simulink model "MultiUAV_DroneShow"  (R2026a)
settings: Solver=ode1  StopTime=74.3333  FixedStep=Ts_sim  MaxStep=0.01  AbsTol=1e-6
PreLoadFcn:
  | setupParams
values from neighbouring files (symbols this model uses):
  arm_duration = 2    [setupParams.m]
  gnss_deny_mask = false(N_uav, 1)    [setupParams.m]
  gnss_err_gain = sqrt(1 - gnss_err_pole^2)    [setupParams.m]
  gnss_err_pole = exp(-Ts_sim / gnss_err_tau)    [setupParams.m]
  gnss_err_seed = reshape(40000 + (1:(N_uav * 3)), N_uav, 3)    [setupParams.m]
  gps_accuracy_rtk_fix = 0.02    [setupParams.m]
  gps_lock_duration = 2    [setupParams.m]
  gravity = 9.81    [setupParams.m]
  hb_period_ticks = mavlink_hb_interval / Ts_sim    (= 100)    [setupParams.m]
  init_positions = init_positions(pad_of, :)    [planShow.m]    (also in setupParams.m = plan.init_positions)
  Kd_pos = repmat([Kd_xy Kd_xy Kd_z], N_uav, 1)    [setupParams.m]
  Kff_pos = Kd_pos    [setupParams.m]
  Kp_pos = repmat([Kp_xy Kp_xy Kp_z], N_uav, 1)    [setupParams.m]
  land_end_time = plan.land_end_time    [packShowUpload.m]    (also in planShow.m = show_flight_duration + land_duration; setupParams.m)
  land_speed = cfg.land_speed    [planShow.m]
  land_start_time = show_flight_duration    [planShow.m]    (also in setupParams.m = plan.land_start_time)
  land_total_duration = land_duration + land_settle    [planShow.m]    (also in setupParams.m = plan.land_total_duration)
  mav_sys_span = 250    [setupParams.m]
  N_uav = 20    [DroneShowExample.m]    (also in packShowUpload.m = cfg.N_uav; planShow.m = cfg.N_uav; setupParams.m = 10)
  num_waypoints = length(upload_times)    [packShowUpload.m]    (also in setupParams.m = pack.num_waypoints)
  rtcm_data_bytes = 180    [setupParams.m]
  rtcm_interval = 1.0    (= 1)    [setupParams.m]
  rtcm_payload_bytes = 4 * 4 * rtk_n_sat    [setupParams.m]
  rtcm_period_ticks = rtcm_interval / Ts_sim    (= 100)    [setupParams.m]
  rtk_amb_l1_base = 1000000 + mod(97 * (1:rtk_n_sat)', 1009)    [setupParams.m]
  rtk_amb_l1_rover = rtk_amb_l1_base + rtk_amb_l1    [setupParams.m]
  rtk_amb_l2_base = 1000000 + mod(89 * (1:rtk_n_sat)', 1009)    [setupParams.m]
  rtk_amb_l2_rover = rtk_amb_l2_base + rtk_amb_l2    [setupParams.m]
  rtk_base_lla = [42.3601, -71.0589, 10]    [setupParams.m]
  rtk_deny_mask = false(N_uav, 1)    [setupParams.m]
  rtk_f1 = 1575.42e6    (= 1575420000)    [setupParams.m]
  rtk_f2 = 1227.60e6    (= 1227600000)    [setupParams.m]
  rtk_fall_slew = -gps_accuracy_standard / reconverge_time    (= -0.3)    [setupParams.m]
  rtk_fix_thresh_l1 = 0.30    (= 0.3)    [setupParams.m]
  rtk_fix_thresh_wl = 0.25    [setupParams.m]
  rtk_inject_enable = double(~skip_preflight | rtk_deny_mask(:)')    [setupParams.m]
  rtk_lambda1 = rtk_c / rtk_f1    (= 0.190293672798)    [setupParams.m]
  rtk_lambda2 = rtk_c / rtk_f2    (= 0.244210213425)    [setupParams.m]
  rtk_lambda_wl = rtk_c / (rtk_f1 - rtk_f2)    (= 0.861918400322)    [setupParams.m]
  rtk_lock_dwell = 2.0    (= 2)    [setupParams.m]
  rtk_los = [cosd(rtk_el) .* sind(rtk_az), cosd(rtk_el) .* cosd(rtk_az), sind(rtk_el)]    [setupParams.m]
  rtk_mean_clk = zeros(2, 1)    [setupParams.m]
  rtk_mean_obs = zeros(2, rtk_n_sat)    [setupParams.m]
  rtk_n_sat = numel(rtk_az)    [setupParams.m]
  rtk_rough_range = pseudoranges(rtk_base_lla, rtk_sat_pos, 'RangeAccuracy', 0)    [setupParams.m]
  rtk_sat_pos = rtk_sat_pos_all(rtk_vis, :)    [setupParams.m]
  rtk_seedm_clk = 9101 + 8 * rtk_n_sat + (0:1)'    [setupParams.m]
  rtk_seedm_l1 = rtk_seedm_p2 + 2 * rtk_n_sat    [setupParams.m]
  rtk_seedm_l2 = rtk_seedm_l1 + 2 * rtk_n_sat    [setupParams.m]
  rtk_seedm_p1 = 9101 + reshape(0:2 * rtk_n_sat - 1, 2, rtk_n_sat)    [setupParams.m]
  rtk_seedm_p2 = rtk_seedm_p1 + 2 * rtk_n_sat    [setupParams.m]
  rtk_sigma_bp = [0, rtk_timeout, rtk_float_timeout]    [setupParams.m]
  rtk_sigma_table = sqrt(max(0, rtk_sigma_tiers.^2 - gps_accuracy_rtk_fix^2))    [setupParams.m]
  rtk_sigma_unfixed = 0.75    [setupParams.m]
  rtk_slip_thresh_l1 = 0.02    [setupParams.m]
  rtk_slip_thresh_wl = 0.10    (= 0.1)    [setupParams.m]
  rtk_status_l1 = 1    [setupParams.m]
  rtk_status_unfixed = 3    [setupParams.m]
  rtk_timeout = 2.5    [setupParams.m]
  rtk_var_clk = rtk_clock_sigma^2 * ones(2, 1)    [setupParams.m]
  rtk_var_l = [rtk_sigma_phase_base^2; rtk_sigma_phase_rover^2] * ones(1, rtk_n_sat)    [setupParams.m]
  rtk_var_p = [rtk_sigma_code_base^2;  rtk_sigma_code_rover^2 ] * ones(1, rtk_n_sat)    [setupParams.m]
  skip_preflight = traj_source == 1    [DroneShowExample.m]    (also in setupParams.m = false)
  st_period_ticks = mavlink_st_interval / Ts_sim    (= 100)    [setupParams.m]
  st_phase_ticks = st_period_ticks / 2    (= 50)    [setupParams.m]
  telemetry_tx_enable = double(~skip_preflight)    [setupParams.m]
  traj_upload_flat = zeros(N_uav*num_waypoints, 7)    [packShowUpload.m]    (also in setupParams.m = pack.traj_upload_flat)
  Ts_sim = cfg.Ts_sim    [packShowUpload.m]    (also in setupParams.m = 0.01)
  uav_loss_seed = 31000 + (1:N_uav)    [setupParams.m]
  uav_mass = 0.1    [setupParams.m]
  upload_duration = (total_packets + N_uav) * Ts_sim * 1.2    [packShowUpload.m]    (also in setupParams.m = pack.upload_duration)
  upload_rate_vec = [1 ./ upload_dt; 1 / upload_dt(end)]    [packShowUpload.m]    (also in setupParams.m = pack.upload_rate_vec)
  upload_request = traj_source == 2    [DroneShowExample.m]
undefined symbols (not defined in the file or in its folder): abort_request, DiscIntNeverNeededParam, doppler, loss_seed, packet_loss_rate, Payload, SystemID, uav_loss_rate
libraries: uavmavlinklib x22, hdlsllib x16, dspsigops x8, simulink x7, matrix_library x4, commchan3 x2, etargetslib x1, uavalgslib x1, sensorinslib x1, slpidlib x1, dspmathops x1, commrandsrc3 x1
(part 1 of 4)
settings Model: Creator=rvalenti  LastModifiedBy=rvalenti
settings DebuggingCC: RTPrefix=warning

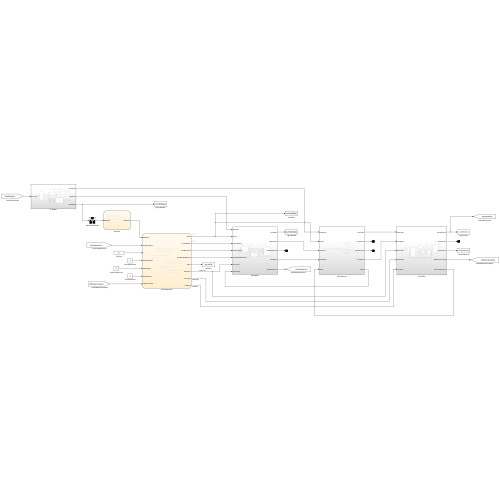
[thumbnail: Simulink's stored preview of the top-level diagram]
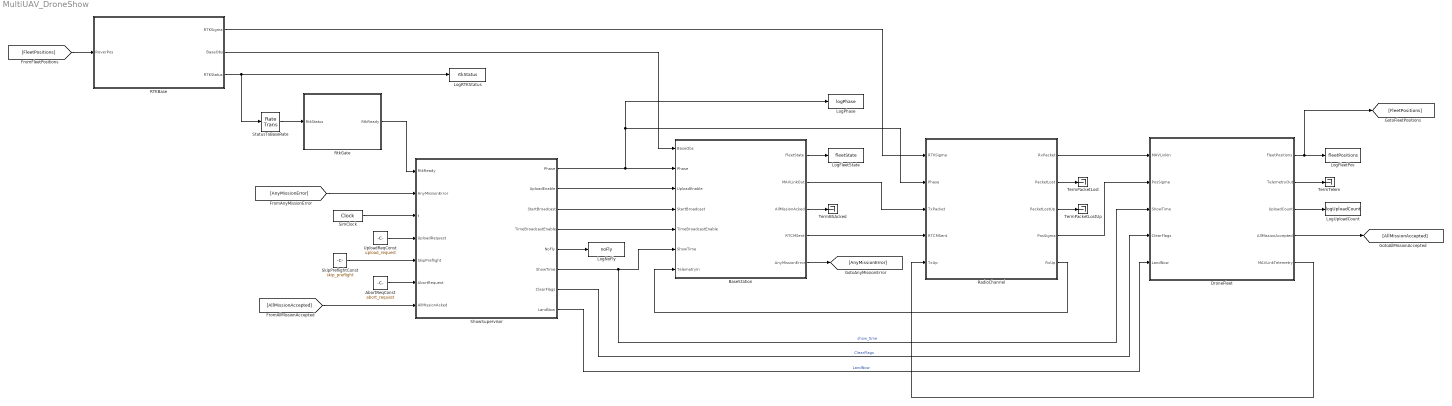
== system MultiUAV_DroneShow ==
  AbortReqConst : Constant  Value=abort_request  OutDataTypeStr=boolean  SampleTime=Ts_sim
  BaseStation : Subsystem
  DroneFleet : Subsystem
  LogFleetPos : ToWorkspace  VariableName=fleetPositions  SaveFormat=Timeseries  SampleTime=-1
  LogFleetState : ToWorkspace  VariableName=fleetState  SaveFormat=Timeseries  SampleTime=-1
  LogNoFly : ToWorkspace  VariableName=noFly  SampleTime=-1
  LogPhase : ToWorkspace  VariableName=logPhase  SaveFormat=Timeseries  SampleTime=Ts_sim
  LogRTKStatus : ToWorkspace  VariableName=rtkStatus  SaveFormat=Timeseries  SampleTime=-1
  LogUploadCount : ToWorkspace  VariableName=logUploadCount  SaveFormat=Timeseries  SampleTime=Ts_sim
  RTKBase : Subsystem
  RadioChannel : Subsystem
  RtkGate : Stateflow chart  TreatAsAtomicUnit=on
  ShowSupervisor : Stateflow chart  TreatAsAtomicUnit=on
      settings: PortSchema="{\"entries\":[{\"content\":{\"sides\":[{\"content\":{\"connectorIds\":[\"In7\",\"In2\",\"In3\",\"In4\",\"In5\",\"In6\",\"In1\"]},\"type\":\"ConnectorPlacement.EquallySpacedRectSide\",\"uuid\":\"11416b01-b04f-4930-8bfb-b8d06603e7e7\"},{\"content\":{\"connectorIds\":[\"Out1\",\"Out3\",\"Out4\",\"Out5\",\"Out8\",\"Out2\",\"Out6\",\"Out7\"],\"side\":\"RIGHT\"},\"type\":\"ConnectorPlacement.EquallySpacedRectSide\",\"uuid\":\"8effc10f-123e-42e7-8478-5d17c541bd6e\"},{\"content\":{\"side\":\"TOP\"},\"type\":\"ConnectorPlacement.EquallySpacedRectSide\",\"uuid\":\"c257d611-a774-4dfa-b469-f119b49a9574\"}]},\"type\":\"ConnectorPlacement.EquallySpacedConnector\",\"uuid\":\"6a641874-f187-4c96-a191-4ddd5039745b\"}],\"packageUris\":[\"http://schema.mathworks.com/mf0/Connector/R2020b\"],\"version\":\"1.0\"}"
  SimClock : DigitalClock  SampleTime=Ts_sim
  SkipPreflightConst : Constant  Value=skip_preflight  OutDataTypeStr=boolean
  StatusToBaseRate : RateTransition  InitialCondition=rtk_status_unfixed
  TermBSAcked : Terminator
  TermPacketLost : Terminator
  TermPacketLostUp : Terminator
  TermTelem : Terminator
  UploadReqConst : Constant  Value=upload_request  OutDataTypeStr=boolean
  wires:
  RTKBase/2(BaseObs) -> BaseStation/1(BaseObs)
  RTKBase/3(RTKStatus) -> StatusToBaseRate/1, LogRTKStatus/1
  StatusToBaseRate/1 -> RtkGate/1(RtkStatus)
  RtkGate/1(RtkReady) -> ShowSupervisor/7(RtkReady)
  [FleetPositions] -> RTKBase/1(RoverPos)
  [AllMissionAccepted] -> ShowSupervisor/1(AllMissionAcked)
  [AnyMissionError] -> ShowSupervisor/2(AnyMissionError)
  SimClock/1 -> ShowSupervisor/3(t)
  UploadReqConst/1 -> ShowSupervisor/4(UploadRequest)
  SkipPreflightConst/1 -> ShowSupervisor/5(SkipPreflight)
  AbortReqConst/1 -> ShowSupervisor/6(AbortRequest)
  ShowSupervisor/1(Phase) -> BaseStation/2(Phase), RadioChannel/2(Phase), LogPhase/1
  ShowSupervisor/2(ShowTime) -> BaseStation/6(ShowTime), DroneFleet/3(ShowTime)  "show_time"
  ShowSupervisor/3(UploadEnable) -> BaseStation/3(UploadEnable)
  ShowSupervisor/4(StartBroadcast) -> BaseStation/4(StartBroadcast)
  ShowSupervisor/5(TimeBroadcastEnable) -> BaseStation/5(TimeBroadcastEnable)
  ShowSupervisor/8(NoFly) -> LogNoFly/1
  ShowSupervisor/6(ClearFlags) -> DroneFleet/4(ClearFlags)  "ClearFlags"
  ShowSupervisor/7(LandNow) -> DroneFleet/5(LandNow)  "LandNow"
  RTKBase/1(RTKSigma) -> RadioChannel/1(RTKSigma)
  BaseStation/2(MAVLinkOut) -> RadioChannel/3(TxPacket)
  BaseStation/1(FleetState) -> LogFleetState/1
  BaseStation/3(AllMissionAcked) -> TermBSAcked/1
  BaseStation/5(AnyMissionError) -> [AnyMissionError]
  BaseStation/4(RTCMSent) -> RadioChannel/4(RTCMSent)
  RadioChannel/2(PacketLost) -> TermPacketLost/1
  RadioChannel/3(PacketLostUp) -> TermPacketLostUp/1
  RadioChannel/1(RxPacket) -> DroneFleet/1(MAVLinkIn)
  RadioChannel/4(PosSigma) -> DroneFleet/2(PosSigma)
  DroneFleet/1(FleetPositions) -> LogFleetPos/1, [FleetPositions]
  DroneFleet/2(TelemetryOut) -> TermTelem/1
  DroneFleet/3(UploadCount) -> LogUploadCount/1
  DroneFleet/4(AllMissionAccepted) -> [AllMissionAccepted]
  RadioChannel/5(RxUp) -> BaseStation/7(TelemetryIn)
  DroneFleet/5(MAVLinkTelemetry) -> RadioChannel/5(TxUp)

== system MultiUAV_DroneShow/BaseStation ==
  BaseObs : Inport
  Phase : Inport  Port=2
  UploadEnable : Inport  Port=3
  StartBroadcast : Inport  Port=4
  TimeBroadcastEnable : Inport  Port=5
  ShowTime : Inport  Port=6
  TelemetryIn : Inport  Port=7
  MissionProtocol : Subsystem
  NumWP_c : Constant  Value=num_waypoints  OutDataTypeStr=uint32
  Receiver : Subsystem
  Transmitter : Subsystem
  UplinkScheduler : Subsystem
  FleetState : Outport
  MAVLinkOut : Outport  Port=2
  AllMissionAcked : Outport  Port=3
  RTCMSent : Outport  Port=4
  AnyMissionError : Outport  Port=5
  wires:
  TelemetryIn/1 -> MissionProtocol/4(TelemetryIn), Receiver/1(TelemetryIn)
  UploadEnable/1 -> MissionProtocol/3(UploadEnable)
  MissionProtocol/5(AllAcked) -> AllMissionAcked/1
  MissionProtocol/3(ItemTarget) -> Transmitter/2(ItemTarget)
  Phase/1 -> MissionProtocol/2(Phase), UplinkScheduler/4(Phase)
  NumWP_c/1 -> MissionProtocol/1(NumWaypoints), Transmitter/5(NumWaypoints)
  Receiver/1(FleetState) -> FleetState/1
  MissionProtocol/1(UploadMode) -> UplinkScheduler/3(UploadMode)
  UplinkScheduler/1(MsgIdx) -> Transmitter/6(MsgIdx)
  MissionProtocol/2(MCTarget) -> Transmitter/1(MCTarget)
  MissionProtocol/4(ItemSeq) -> Transmitter/3(ItemSeq)
  MissionProtocol/6(AnyError) -> AnyMissionError/1
  MissionProtocol/7(LinIdx) -> Transmitter/4(LinIdx)
  StartBroadcast/1 -> UplinkScheduler/1(StartBroadcast)
  TimeBroadcastEnable/1 -> UplinkScheduler/2(TimeBroadcastEnable)
  UplinkScheduler/2(MCEnable) -> Transmitter/7(MCEnable)
  UplinkScheduler/3(CLEnable) -> Transmitter/8(CLEnable)
  UplinkScheduler/4(RTCMSend) -> RTCMSent/1, Transmitter/11(RTCMSend)
  ShowTime/1 -> Transmitter/9(ShowTime)
  BaseObs/1 -> Transmitter/10(BaseObs)
  Transmitter/1(MAVLinkOut) -> MAVLinkOut/1

== system MultiUAV_DroneShow/DroneFleet ==
  MAVLinkIn : Inport
  PosSigma : Inport  Port=2
  ShowTime : Inport  Port=3
  ClearFlags : Inport  Port=4
  LandNow : Inport  Port=5
  FlightDynamics : Subsystem
  MissionStatus : Subsystem
  Navigation : Subsystem
  OnboardBuffer : DataStoreMemory  DataStoreName=OnboardBuffer  InitialValue=zeros(N_uav*num_waypoints,3)  ShowAdditionalParam=off  OutDataTypeStr=double  Dimensions=[N_uav*num_waypoints, 3]
  PositionController : Subsystem
  ReceivedFlags : DataStoreMemory  DataStoreName=ReceivedFlags  InitialValue=zeros(N_uav*num_waypoints,1,'uint8')  ShowAdditionalParam=off  OutDataTypeStr=uint8  Dimensions=[N_uav*num_waypoints, 1]
  Receiver : Subsystem
  SetpointGenerator : Subsystem
  Transmitter : Subsystem
  FleetPositions : Outport
  TelemetryOut : Outport  Port=2
  UploadCount : Outport  Port=3
  AllMissionAccepted : Outport  Port=4
  MAVLinkTelemetry : Outport  Port=5
  wires:
  ShowTime/1 -> SetpointGenerator/2(ShowTime)  "show_time"
  Transmitter/1(TelemetryBus) -> TelemetryOut/1
  Navigation/3(MeasPos) -> Transmitter/6(MeasPos), PositionController/4(EstPos)
  Navigation/2(EstOri) -> PositionController/6(EstOri)
  MissionStatus/1(UploadCount) -> UploadCount/1
  MissionStatus/4(AckTrigger) -> Transmitter/2(AckTrigger)
  MissionStatus/2(AllAccepted) -> AllMissionAccepted/1
  MissionStatus/3(MissionFlags) -> Transmitter/1(MissionFlags)
  Transmitter/2(MAVLinkBytes) -> MAVLinkTelemetry/1
  PosSigma/1 -> Navigation/4(PosSigma)
  FlightDynamics/3(TrueOri) -> Navigation/3(TrueOri)
  Receiver/1(RxStatus) -> Transmitter/3(RxStatus), MissionStatus/1(RxStatus)
  Receiver/2(RxTargetSys) -> Transmitter/4(RxTargetSys)
  PositionController/4(Thrust) -> FlightDynamics/4(CmdThrust)
  PositionController/3(YawRate) -> FlightDynamics/3(CmdYawRate)
  Navigation/1(EstVel) -> Transmitter/5(EstVel), PositionController/5(EstVel)
  PositionController/2(Pitch) -> FlightDynamics/2(CmdPitch)
  PositionController/1(Roll) -> FlightDynamics/1(CmdRoll)
  ClearFlags/1 -> Receiver/1(ClearFlags)
  MAVLinkIn/1 -> Receiver/2(MAVLinkBytes)
  SetpointGenerator/2(CmdVel) -> PositionController/2(TargetVel)
  SetpointGenerator/3(CmdYaw) -> PositionController/3(TargetYaw)
  FlightDynamics/1(TruePos) -> FleetPositions/1, Navigation/1(TruePos)
  SetpointGenerator/1(CmdPos) -> PositionController/1(TargetPos)
  LandNow/1 -> SetpointGenerator/1(LandNow)
  FlightDynamics/2(TrueVel) -> Navigation/2(TrueVel)

== system MultiUAV_DroneShow/RTKBase ==
  RoverPos : Inport
  BaseResiduals : Subsystem  TreatAsAtomicUnit=on
  LogRTKBaseline : ToWorkspace  VariableName=rtkBaseline  SampleTime=-1
  ObservableSource : Subsystem  Description=Fills GNSSObservableBus for RTKEngine. Simulated generates observables from the flown rover position; Measured plays back a recorded base/rover pair. The engine downstream is the same block either way -- rtk_obs_source selects.  Variant=on
  RTKEngine : Subsystem
  SigmaToBaseRate : RateTransition  InitialCondition=rtk_sigma_unfixed
  SplitBaseObs : BusSelector  OutputSignals=P1,P2,L1,L2,Valid
  TermRTKDiag : Terminator
  ToBaseRate : RateTransition
  RTKSigma : Outport
  BaseObs : Outport  Port=2
  RTKStatus : Outport  Port=3
  wires:
  RTKEngine/2(Sigma) -> SigmaToBaseRate/1
  RTKEngine/3(Status) -> RTKStatus/1
  RTKEngine/4(Diag) -> TermRTKDiag/1
  RoverPos/1 -> ObservableSource/1(RoverPos)
  ObservableSource/1(Obs) -> SplitBaseObs/1, RTKEngine/1(Obs)  "GNSSObservables"
  RTKEngine/1(Baseline) -> LogRTKBaseline/1
  ToBaseRate/1 -> BaseObs/1
  SplitBaseObs/1 -> BaseResiduals/1(P1)  "<P1>"
  SplitBaseObs/2 -> BaseResiduals/2(P2)  "<P2>"
  SplitBaseObs/3 -> BaseResiduals/3(L1)  "<L1>"
  SplitBaseObs/4 -> BaseResiduals/4(L2)  "<L2>"
  SplitBaseObs/5 -> BaseResiduals/5(Valid)  "<Valid>"
  BaseResiduals/1(BaseObs) -> ToBaseRate/1
  SigmaToBaseRate/1 -> RTKSigma/1

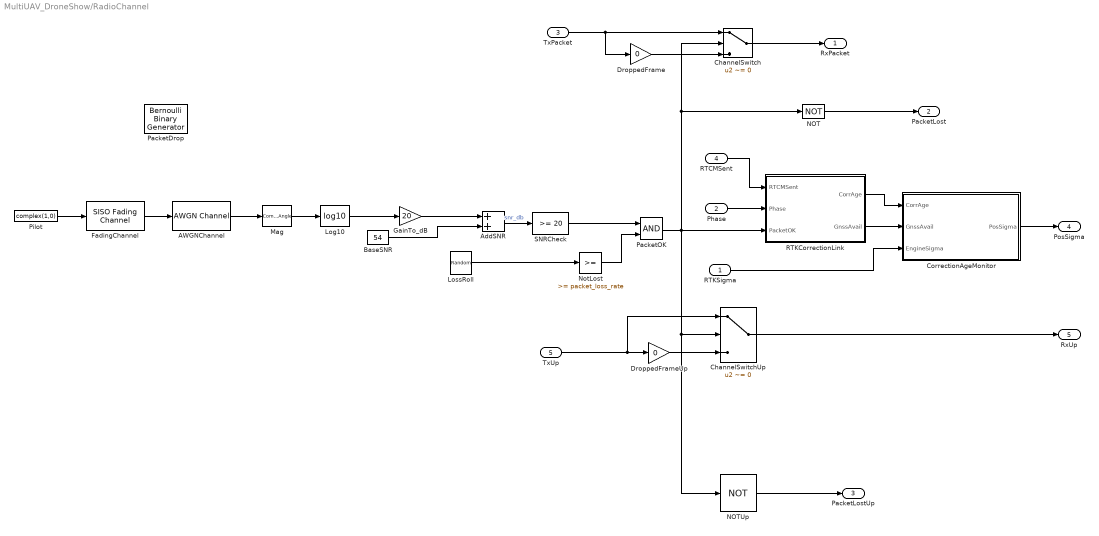
== system MultiUAV_DroneShow/RadioChannel ==
  RTKSigma : Inport
  Phase : Inport  Port=2
  TxPacket : Inport  Port=3
  RTCMSent : Inport  Port=4
  TxUp : Inport  Port=5
  AWGNChannel : commchan3/AWGN Channel  LegacyMode=off  NoiseMethod="Signal to noise ratio  (SNR)"  noiseMode="Signal to noise ratio  (SNR)"  EbNo=10  EsNo=10  SNR=54  BitsPerSymbol=1  SignalPower=1  SpecifySymbolPeriod=off  SamplesPerSymbol=1  SymbolPeriod=1  VarianceSource=Parameter  Variance=1  RandomStream=Global stream  Seed=67  SimulateUsing=Code generation
  AddSNR : Sum
  BaseSNR : Constant  Value=54
  ChannelSwitch : Switch  Criteria=u2 ~= 0  SaturateOnIntegerOverflow=off  InputSameDT=off
  ChannelSwitchUp : Switch  Criteria=u2 ~= 0
  CorrectionAgeMonitor : Subsystem
  DroppedFrame : Gain  Gain=0  OutDataTypeStr=Inherit: Same as input
  DroppedFrameUp : Gain  Gain=0  OutDataTypeStr=Inherit: Same as input
  FadingChannel : commchan3/SISO Fading Channel  InheritSampleRate=off  SampleRate=1/Ts_sim  PathDelays=[0 5e-8]  AveragePathGains=[0 -10]  NormalizePathGains=on  FadingDistribution=Rician  KFactor=10  DirectPathDopplerShift=0  DirectPathInitialPhase=0  MaximumDopplerShift=9  DopplerSpectrum=doppler('Jakes')  RandomStream=mt19937ar with seed  Seed=73  PathGainsOutputPort=off  ChannelFilterDelayOutputPort=off  SimulateUsing=Code generation  Visualization=Off  PathsForDopplerDisplay=1  SamplesToDisplay=25%
  GainTo_dB : Gain  Gain=20
  Log10 : Math  Operator=log10
  LossRoll : UniformRandomNumber  Minimum=0  Seed=loss_seed  SampleTime=Ts_sim
  Mag : ComplexToMagnitudeAngle  Output=Magnitude
  NOT : Logic  Operator=NOT  AllPortsSameDT=off  OutDataTypeStr=boolean
  NOTUp : Logic  Operator=NOT
  NotLost : hdlsllib/Logic and Bit Operations/Compare To Constant  relop=>=  const=packet_loss_rate  OutDataTypeStr=boolean
  PacketOK : Logic
  Pilot : Constant  Value=complex(1,0)  OutDataTypeStr=double
  RTKCorrectionLink : Subsystem
  SNRCheck : simulink/Logic and Bit Operations/Compare To Constant  relop=>=  const=20  OutDataTypeStr=boolean
  RxPacket : Outport
  PacketLost : Outport  Port=2
  PacketLostUp : Outport  Port=3
  PosSigma : Outport  Port=4
  RxUp : Outport  Port=5
  PacketDrop : commrandsrc3/Bernoulli Binary Generator  IOType=siggen  ProbabilityOfZero=1 - packet_loss_rate  SeedSource=Auto  Seed=0  SampleTime=Ts_sim  SamplesPerFrame=1  OutputDataType=boolean  SimulateUsing=Interpreted execution
      settings: LibrarySourceBlock=|
      | commgenrandsrc3/Bernoulli Binary
      | Generator
  wires:
  RTKSigma/1 -> CorrectionAgeMonitor/3(EngineSigma)
  CorrectionAgeMonitor/1(PosSigma) -> PosSigma/1
  NOTUp/1 -> PacketLostUp/1
  ChannelSwitchUp/1 -> RxUp/1
  RTKCorrectionLink/1(CorrAge) -> CorrectionAgeMonitor/1(CorrAge)
  RTKCorrectionLink/2(GnssAvail) -> CorrectionAgeMonitor/2(GnssAvail)
  NOT/1 -> PacketLost/1
  ChannelSwitch/1 -> RxPacket/1
  DroppedFrameUp/1 -> ChannelSwitchUp/3
  PacketOK/1 -> RTKCorrectionLink/3(PacketOK), NOT/1, ChannelSwitch/2, ChannelSwitchUp/2, NOTUp/1
  Phase/1 -> RTKCorrectionLink/2(Phase)
  RTCMSent/1 -> RTKCorrectionLink/1(RTCMSent)
  NotLost/1 -> PacketOK/2
  DroppedFrame/1 -> ChannelSwitch/3
  SNRCheck/1 -> PacketOK/1
  LossRoll/1 -> NotLost/1
  AddSNR/1 -> SNRCheck/1  "snr_db"
  BaseSNR/1 -> AddSNR/2
  TxPacket/1 -> ChannelSwitch/1, DroppedFrame/1
  GainTo_dB/1 -> AddSNR/1
  Mag/1 -> Log10/1
  Log10/1 -> GainTo_dB/1
  FadingChannel/1 -> AWGNChannel/1
  Pilot/1 -> FadingChannel/1
  TxUp/1 -> ChannelSwitchUp/1, DroppedFrameUp/1
  AWGNChannel/1 -> Mag/1

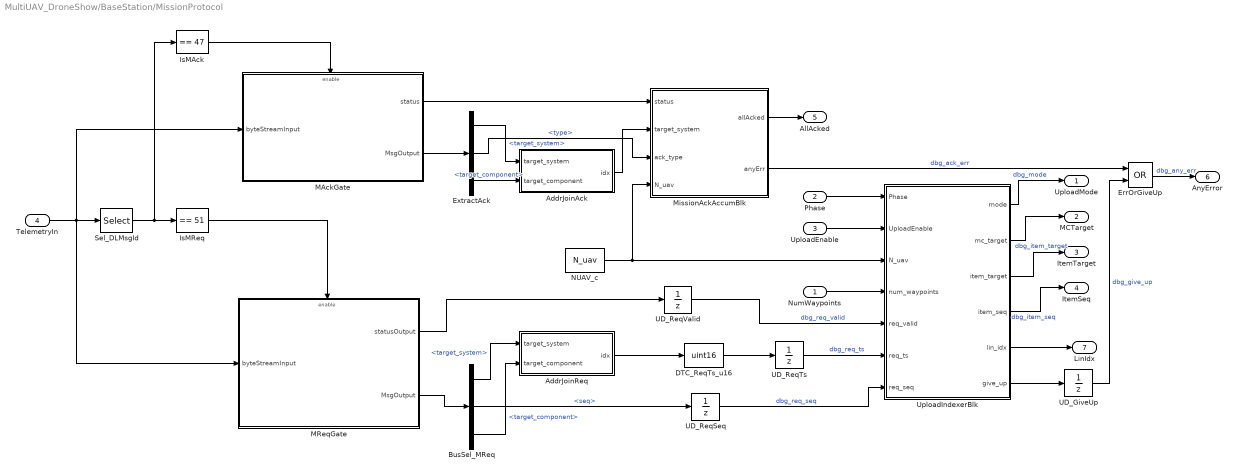
== system MultiUAV_DroneShow/BaseStation/MissionProtocol ==
  NumWaypoints : Inport
  Phase : Inport  Port=2
  UploadEnable : Inport  Port=3
  TelemetryIn : Inport  Port=4
  AddrJoinAck : Subsystem
  AddrJoinReq : Subsystem
  BusSel_MReq : BusSelector  OutputSignals=Payload.target_system,Payload.seq,Payload.target_component
  DTC_ReqTs_u16 : DataTypeConversion  OutDataTypeStr=uint16
  ErrOrGiveUp : Logic  Operator=OR  AllPortsSameDT=off  OutDataTypeStr=boolean
  ExtractAck : BusSelector  OutputSignals=Payload.target_system,Payload.type,Payload.target_component
  IsMAck : simulink/Logic and Bit Operations/Compare To Constant  relop===  const=47  OutDataTypeStr=boolean
  IsMReq : simulink/Logic and Bit Operations/Compare To Constant  relop===  const=51  OutDataTypeStr=boolean
  MAckGate : Subsystem
  MReqGate : Subsystem
  MissionAckAccumBlk : Subsystem
  NUAV_c : Constant  Value=N_uav  OutDataTypeStr=uint32
  Sel_DLMsgId : Selector  NumberOfDimensions=2  InputPortWidth=3  IndexOptions=Index vector (dialog),Index vector (dialog)  Indices=1,8  OutputSizes=1,1
  UD_GiveUp : UnitDelay  InitialCondition=false  SampleTime=Ts_sim
  UD_ReqSeq : UnitDelay  InitialCondition=uint16(0)  SampleTime=Ts_sim
  UD_ReqTs : UnitDelay  InitialCondition=uint8(0)  SampleTime=Ts_sim
  UD_ReqValid : UnitDelay  InitialCondition=false  SampleTime=Ts_sim
  UploadIndexerBlk : Subsystem
  UploadMode : Outport
  MCTarget : Outport  Port=2
  ItemTarget : Outport  Port=3
  ItemSeq : Outport  Port=4
  AllAcked : Outport  Port=5
  AnyError : Outport  Port=6
  LinIdx : Outport  Port=7
  wires:
  Phase/1 -> UploadIndexerBlk/1(Phase)
  AddrJoinAck/1(idx) -> MissionAckAccumBlk/2(target_system)
  TelemetryIn/1 -> MAckGate/1(byteStreamInput), MReqGate/1(byteStreamInput), Sel_DLMsgId/1
  Sel_DLMsgId/1 -> IsMAck/1, IsMReq/1
  IsMAck/1 -> MAckGate/Enable
  MAckGate/2(MsgOutput) -> ExtractAck/1
  UploadIndexerBlk/5(lin_idx) -> LinIdx/1
  UD_ReqTs/1 -> UploadIndexerBlk/6(req_ts)  "dbg_req_ts"
  IsMReq/1 -> MReqGate/Enable
  MAckGate/1(status) -> MissionAckAccumBlk/1(status)
  MReqGate/2(MsgOutput) -> BusSel_MReq/1
  MReqGate/1(statusOutput) -> UD_ReqValid/1
  BusSel_MReq/1 -> AddrJoinReq/1(target_system)  "<target_system>"
  ExtractAck/1 -> AddrJoinAck/1(target_system)  "<target_system>"
  ErrOrGiveUp/1 -> AnyError/1  "dbg_any_err"
  DTC_ReqTs_u16/1 -> UD_ReqTs/1
  BusSel_MReq/2 -> UD_ReqSeq/1  "<seq>"
  ExtractAck/2 -> MissionAckAccumBlk/3(ack_type)  "<type>"
  BusSel_MReq/3 -> AddrJoinReq/2(target_component)  "<target_component>"
  ExtractAck/3 -> AddrJoinAck/2(target_component)  "<target_component>"
  NUAV_c/1 -> MissionAckAccumBlk/4(N_uav), UploadIndexerBlk/3(N_uav)
  AddrJoinReq/1(idx) -> DTC_ReqTs_u16/1
  MissionAckAccumBlk/1(allAcked) -> AllAcked/1
  MissionAckAccumBlk/2(anyErr) -> ErrOrGiveUp/1  "dbg_ack_err"
  UD_ReqValid/1 -> UploadIndexerBlk/5(req_valid)  "dbg_req_valid"
  UD_ReqSeq/1 -> UploadIndexerBlk/7(req_seq)  "dbg_req_seq"
  NumWaypoints/1 -> UploadIndexerBlk/4(num_waypoints)
  UploadEnable/1 -> UploadIndexerBlk/2(UploadEnable)
  UploadIndexerBlk/1(mode) -> UploadMode/1  "dbg_mode"
  UploadIndexerBlk/2(mc_target) -> MCTarget/1
  UploadIndexerBlk/3(item_target) -> ItemTarget/1  "dbg_item_target"
  UploadIndexerBlk/4(item_seq) -> ItemSeq/1  "dbg_item_seq"
  UploadIndexerBlk/6(give_up) -> UD_GiveUp/1
  UD_GiveUp/1 -> ErrOrGiveUp/2  "dbg_give_up"

== system MultiUAV_DroneShow/BaseStation/Receiver ==
  TelemetryIn : Inport
  AssignTelemetry : Assignment  NumberOfDimensions=2  IndexOptions=Index vector (port),Assign all  Indices=1  OutputSizes=N_uav,6
  DTC_SysIdx : DataTypeConversion  OutDataTypeStr=uint32
  DTC_TelData : DataTypeConversion  OutDataTypeStr=double
  Deser_Telemetry : uavmavlinklib/MAVLink Deserializer  dialectSource=Select from standard MAVLink dialects  dialect=common.xml  dialectCustom=common.xml  version=2  messageType=LOCAL_POSITION_NED  inputDataLength=off  SystemIDFilter=off  systemID=1  ComponentIDFilter=off  componentID=1  queueMsg=off  queueMsgSize=50  dropNum=off
  ExtractSystemID : BusSelector  OutputSignals=SystemID
  ExtractTelemetry : BusSelector  OutputSignals=Payload.x,Payload.y,Payload.z,Payload.vx,Payload.vy,Payload.vz
  MuxTelemetry : Mux  Inputs=6
  ReshapeTelData : Reshape  OutputDimensionality=Customize  OutputDimensions=[1 6]
  SwTelTable : Switch  Criteria=u2 > Threshold  Threshold=0.5  SaturateOnIntegerOverflow=off  InputSameDT=off
  SysIdxClamp : Saturate  UpperLimit=N_uav  LowerLimit=1
  SysIdxInRange : simulink/Logic and Bit Operations/Interval Test  IntervalClosedRight=on  uplimit=N_uav  IntervalClosedLeft=on  lowlimit=1  OutDataTypeStr=boolean
  TelMemory : UnitDelay  InitialCondition=zeros(N_uav, 6)  SampleTime=Ts_sim
  TermTelStatus : Terminator
  FleetState : Outport
  wires:
  TelemetryIn/1 -> Deser_Telemetry/1
  Deser_Telemetry/1 -> TermTelStatus/1
  Deser_Telemetry/2 -> ExtractSystemID/1, ExtractTelemetry/1
  ExtractTelemetry/3 -> MuxTelemetry/3  "<z>"
  ExtractTelemetry/1 -> MuxTelemetry/1  "<x>"
  ExtractTelemetry/4 -> MuxTelemetry/4  "<vx>"
  ExtractTelemetry/2 -> MuxTelemetry/2  "<y>"
  ExtractTelemetry/5 -> MuxTelemetry/5  "<vy>"
  ExtractTelemetry/6 -> MuxTelemetry/6  "<vz>"
  MuxTelemetry/1 -> DTC_TelData/1
  ExtractSystemID/1 -> DTC_SysIdx/1  "<SystemID>"
  DTC_TelData/1 -> ReshapeTelData/1
  DTC_SysIdx/1 -> SysIdxInRange/1, SysIdxClamp/1
  TelMemory/1 -> SwTelTable/3, AssignTelemetry/1
  ReshapeTelData/1 -> AssignTelemetry/2
  SysIdxClamp/1 -> AssignTelemetry/3
  AssignTelemetry/1 -> SwTelTable/1
  SysIdxInRange/1 -> SwTelTable/2
  SwTelTable/1 -> FleetState/1, TelMemory/1

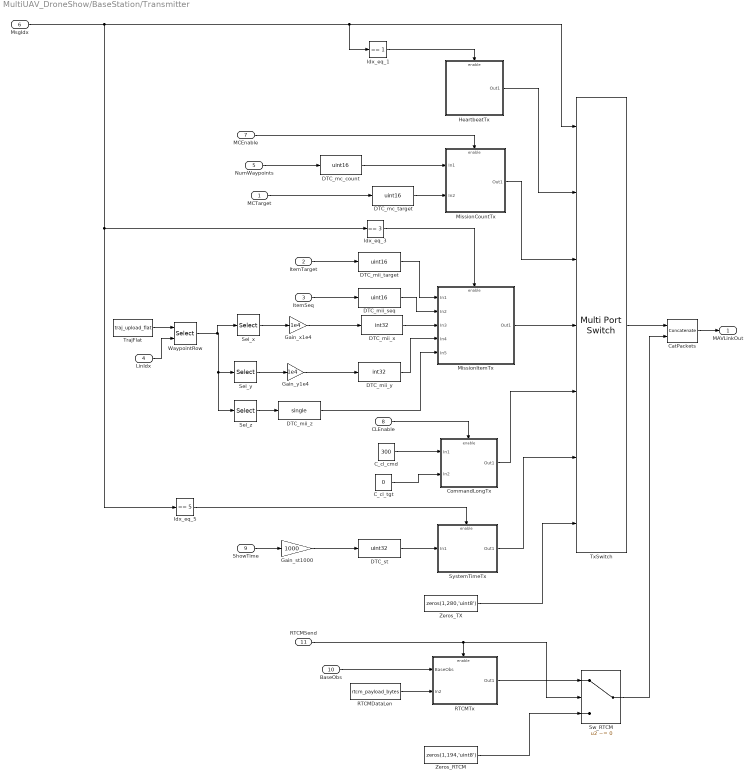
== system MultiUAV_DroneShow/BaseStation/Transmitter ==
  MCTarget : Inport
  ItemTarget : Inport  Port=2
  ItemSeq : Inport  Port=3
  LinIdx : Inport  Port=4
  NumWaypoints : Inport  Port=5
  MsgIdx : Inport  Port=6
  MCEnable : Inport  Port=7
  CLEnable : Inport  Port=8
  ShowTime : Inport  Port=9
  BaseObs : Inport  Port=10
  RTCMSend : Inport  Port=11
  C_cl_cmd : Constant  Value=300  OutDataTypeStr=uint16
  C_cl_tgt : Constant  Value=0  OutDataTypeStr=uint8
  CatPackets : Concatenate
  CommandLongTx : Subsystem
  DTC_mc_count : DataTypeConversion  OutDataTypeStr=uint16
  DTC_mc_target : DataTypeConversion  OutDataTypeStr=uint16
  DTC_mii_seq : DataTypeConversion  OutDataTypeStr=uint16
  DTC_mii_target : DataTypeConversion  OutDataTypeStr=uint16
  DTC_mii_x : DataTypeConversion  OutDataTypeStr=int32
  DTC_mii_y : DataTypeConversion  OutDataTypeStr=int32
  DTC_mii_z : DataTypeConversion  OutDataTypeStr=single
  DTC_st : DataTypeConversion  OutDataTypeStr=uint32
  Gain_st1000 : Gain  Gain=1000
  Gain_x1e4 : Gain  Gain=1e4
  Gain_y1e4 : Gain  Gain=1e4
  HeartbeatTx : Subsystem
  Idx_eq_1 : hdlsllib/Logic and Bit Operations/Compare To Constant  relop===  const=1  OutDataTypeStr=boolean
  Idx_eq_3 : hdlsllib/Logic and Bit Operations/Compare To Constant  relop===  const=3  OutDataTypeStr=boolean
  Idx_eq_5 : hdlsllib/Logic and Bit Operations/Compare To Constant  relop===  const=5  OutDataTypeStr=boolean
  MissionCountTx : Subsystem
  MissionItemTx : Subsystem
  RTCMDataLen : Constant  Value=rtcm_payload_bytes  OutDataTypeStr=uint8
  RTCMTx : Subsystem
  Sel_x : Selector  IndexOptions=Index vector (dialog)  Indices=1  OutputSizes=1
  Sel_y : Selector  IndexOptions=Index vector (dialog)  Indices=2  OutputSizes=1
  Sel_z : Selector  IndexOptions=Index vector (dialog)  Indices=3  OutputSizes=1
  Sw_RTCM : Switch  Criteria=u2 ~= 0
  SystemTimeTx : Subsystem
  TrajFlat : Constant  Value=traj_upload_flat  OutDataTypeStr=double
  TxSwitch : MultiPortSwitch  Inputs=6
  WaypointRow : Selector  NumberOfDimensions=2  InputPortWidth=3  IndexOptions=Index vector (port),Select all  Indices=1,1  OutputSizes=1,7
  Zeros_RTCM : Constant  Value=zeros(1,194,'uint8')  OutDataTypeStr=uint8
  Zeros_TX : Constant  Value=zeros(1,280,'uint8')  OutDataTypeStr=uint8
  MAVLinkOut : Outport
  wires:
  Sel_y/1 -> Gain_y1e4/1
  Sw_RTCM/1 -> CatPackets/2
  TrajFlat/1 -> WaypointRow/1
  WaypointRow/1 -> Sel_z/1, Sel_y/1, Sel_x/1
  C_cl_cmd/1 -> CommandLongTx/1(In1)
  CLEnable/1 -> CommandLongTx/Enable
  LinIdx/1 -> WaypointRow/2
  Sel_z/1 -> DTC_mii_z/1
  Sel_x/1 -> Gain_x1e4/1
  MissionItemTx/1(Out1) -> TxSwitch/4
  BaseObs/1 -> RTCMTx/1(BaseObs)
  NumWaypoints/1 -> DTC_mc_count/1
  MCTarget/1 -> DTC_mc_target/1
  ShowTime/1 -> Gain_st1000/1
  MsgIdx/1 -> Idx_eq_3/1, Idx_eq_5/1, Idx_eq_1/1, TxSwitch/1
  ItemTarget/1 -> DTC_mii_target/1
  RTCMSend/1 -> RTCMTx/Enable, Sw_RTCM/2
  MCEnable/1 -> MissionCountTx/Enable
  ItemSeq/1 -> DTC_mii_seq/1
  DTC_mii_x/1 -> MissionItemTx/3(In3)
  Gain_x1e4/1 -> DTC_mii_x/1
  RTCMTx/1(Out1) -> Sw_RTCM/1
  DTC_mii_target/1 -> MissionItemTx/1(In1)
  Gain_y1e4/1 -> DTC_mii_y/1
  DTC_mii_z/1 -> MissionItemTx/5(In5)
  DTC_mc_target/1 -> MissionCountTx/2(In2)
  Gain_st1000/1 -> DTC_st/1
  Idx_eq_1/1 -> HeartbeatTx/Enable
  DTC_mc_count/1 -> MissionCountTx/1(In1)
  Zeros_TX/1 -> TxSwitch/7
  MissionCountTx/1(Out1) -> TxSwitch/3
  Idx_eq_3/1 -> MissionItemTx/Enable
  DTC_mii_seq/1 -> MissionItemTx/2(In2)
  DTC_mii_y/1 -> MissionItemTx/4(In4)
  C_cl_tgt/1 -> CommandLongTx/2(In2)
  Idx_eq_5/1 -> SystemTimeTx/Enable
  DTC_st/1 -> SystemTimeTx/1(In1)
  RTCMDataLen/1 -> RTCMTx/2(In2)
  HeartbeatTx/1(Out1) -> TxSwitch/2
  CommandLongTx/1(Out1) -> TxSwitch/5
  SystemTimeTx/1(Out1) -> TxSwitch/6
  Zeros_RTCM/1 -> Sw_RTCM/3
  TxSwitch/1 -> CatPackets/1
  CatPackets/1 -> MAVLinkOut/1

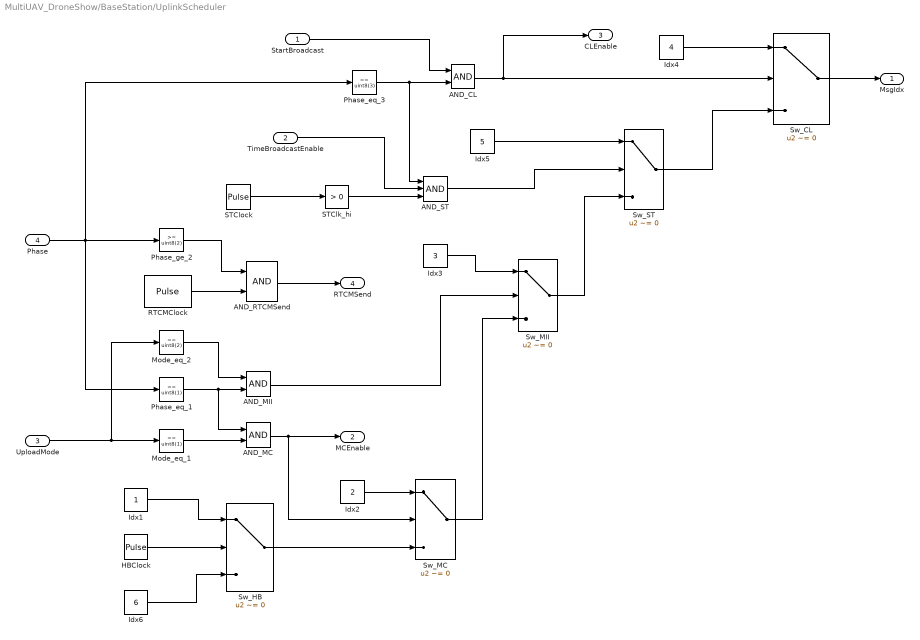
== system MultiUAV_DroneShow/BaseStation/UplinkScheduler ==
  StartBroadcast : Inport
  TimeBroadcastEnable : Inport  Port=2
  UploadMode : Inport  Port=3
  Phase : Inport  Port=4
  AND_CL : Logic
  AND_MC : Logic
  AND_MII : Logic
  AND_RTCMSend : Logic  AllPortsSameDT=off  OutDataTypeStr=boolean
  AND_ST : Logic  Inputs=3
  HBClock : DiscretePulseGenerator  Period=hb_period_ticks  SampleTime=Ts_sim
  Idx1 : Constant  OutDataTypeStr=double
  Idx2 : Constant  Value=2  OutDataTypeStr=double
  Idx3 : Constant  Value=3  OutDataTypeStr=double
  Idx4 : Constant  Value=4  OutDataTypeStr=double
  Idx5 : Constant  Value=5  OutDataTypeStr=double
  Idx6 : Constant  Value=6  OutDataTypeStr=double
  Mode_eq_1 : hdlsllib/Logic and Bit Operations/Compare To Constant  relop===  const=uint8(1)  OutDataTypeStr=boolean
  Mode_eq_2 : hdlsllib/Logic and Bit Operations/Compare To Constant  relop===  const=uint8(2)  OutDataTypeStr=boolean
  Phase_eq_1 : hdlsllib/Logic and Bit Operations/Compare To Constant  relop===  const=uint8(1)  OutDataTypeStr=boolean
  Phase_eq_3 : hdlsllib/Logic and Bit Operations/Compare To Constant  relop===  const=uint8(3)  OutDataTypeStr=boolean
  Phase_ge_2 : hdlsllib/Logic and Bit Operations/Compare To Constant  relop=>=  const=uint8(2)  OutDataTypeStr=boolean
  RTCMClock : DiscretePulseGenerator  Period=rtcm_period_ticks  SampleTime=Ts_sim
  STClk_hi : hdlsllib/Logic and Bit Operations/Compare To Constant  relop=>  const=0  OutDataTypeStr=boolean
  STClock : DiscretePulseGenerator  Period=st_period_ticks  PhaseDelay=st_phase_ticks  SampleTime=Ts_sim
  Sw_CL : Switch  Criteria=u2 ~= 0
  Sw_HB : Switch  Criteria=u2 ~= 0
  Sw_MC : Switch  Criteria=u2 ~= 0
  Sw_MII : Switch  Criteria=u2 ~= 0
  Sw_ST : Switch  Criteria=u2 ~= 0
  MsgIdx : Outport
  MCEnable : Outport  Port=2
  CLEnable : Outport  Port=3
  RTCMSend : Outport  Port=4
  wires:
  RTCMClock/1 -> AND_RTCMSend/2
  Phase/1 -> Phase_ge_2/1, Phase_eq_3/1, Phase_eq_1/1
  Mode_eq_1/1 -> AND_MC/2
  UploadMode/1 -> Mode_eq_1/1, Mode_eq_2/1
  Phase_eq_1/1 -> AND_MII/2, AND_MC/1
  Phase_ge_2/1 -> AND_RTCMSend/1
  Idx2/1 -> Sw_MC/1
  Mode_eq_2/1 -> AND_MII/1
  TimeBroadcastEnable/1 -> AND_ST/2
  Idx1/1 -> Sw_HB/1
  HBClock/1 -> Sw_HB/2
  Idx6/1 -> Sw_HB/3
  STClock/1 -> STClk_hi/1
  AND_RTCMSend/1 -> RTCMSend/1
  AND_CL/1 -> Sw_CL/2, CLEnable/1
  AND_MII/1 -> Sw_MII/2
  AND_MC/1 -> Sw_MC/2, MCEnable/1
  Sw_HB/1 -> Sw_MC/3
  Sw_MII/1 -> Sw_ST/3
  Phase_eq_3/1 -> AND_ST/1, AND_CL/2
  STClk_hi/1 -> AND_ST/3
  Idx3/1 -> Sw_MII/1
  Sw_MC/1 -> Sw_MII/3
  Idx5/1 -> Sw_ST/1
  AND_ST/1 -> Sw_ST/2
  Idx4/1 -> Sw_CL/1
  Sw_ST/1 -> Sw_CL/3
  Sw_CL/1 -> MsgIdx/1
  StartBroadcast/1 -> AND_CL/1

== system MultiUAV_DroneShow/DroneFleet/FlightDynamics ==
  CmdRoll : Inport
  CmdPitch : Inport  Port=2
  CmdYawRate : Inport  Port=3
  CmdThrust : Inport  Port=4
  Bus Selector : BusSelector  OutputSignals=WorldPosition,WorldVelocity,EulerZYX
  ControlBus : BusCreator  Inputs=4  OutDataTypeStr=Bus: MultirotorGuidanceControlBus  NonVirtualBus=on
  EnvBus : BusCreator  Inputs=1  OutDataTypeStr=Bus: MultirotorGuidanceEnvironmentBus  NonVirtualBus=on
  Gravity : Constant  Value=gravity * ones(1, N_uav)
  GuidanceModel : uavalgslib/Multi-Instance Guidance Model  ModelType=MultirotorGuidance  NumInstances=N_uav  SpecifiedDataType=double  SimulateUsing=Code generation  InitialWorldPositionMultirotor=init_positions'  InitialWorldVelocityMultirotor=zeros(3, N_uav)  InitialEulerZYXMultirotor=zeros(3, N_uav)  InitialBodyAngularRateRPYMultirotor=zeros(3, N_uav)  InitialThrustMultirotor=0.1 * gravity * ones(1, N_uav)  InitialNorthFixedWing=[0 0 0 0 0]  InitialEastFixedWing=[0 0 0 0 0]  InitialHeightFixedWing=[0 0 0 0 0]  InitialAirSpeedFixedWing=[0 0 0 0 0]  InitialHeadingAngleFixedWing=[0 0 0 0 0]  InitialFlightPathAngleFixedWing=[0 0 0 0 0]  InitialRollAngleFixedWing=[0 0 0 0 0]  InitialRollAngleRateFixedWing=[0 0 0 0 0]  PDRollMultirotor=repmat([3402.97, 116.67], N_uav, 1)  PDPitchMultirotor=repmat([3402.97, 116.67], N_uav, 1)  PYawRateMultirotor=200 * ones(N_uav, 1)  PThrustMultirotor=200 * ones(N_uav, 1)  MassMultirotor=0.1 * ones(N_uav, 1)  PHeightFixedWing=[3.9; 3.9; 3.9; 3.9; 3.9]  PHeadingAngleFixedWing=[3.9; 3.9; 3.9; 3.9; 3.9]  PFlightPathAngleFixedWing=[39; 39; 39; 39; 39]  PDRollFixedWing=[3402.97 116.67; 3402.97 116.67; 3402.97 116.67; 3402.97 116.67; 3402.97 116.67]  PAirSpeedFixedWing=[1; 1; 1; 1; 1]  FlightPathAngleLimitsFixedWing=[-pi/2 pi/2; -pi/2 pi/2; -pi/2 pi/2; -pi/2 pi/2; -pi/2 pi/2]  StateBusName='MultirotorGuidanceStateBus'  ControlBusName='MultirotorGuidanceControlBus'  EnvironmentBusName='MultirotorGuidanceEnvironmentBus'  DataType=double
      link override ControlSignalSpecification: OutDataTypeStr=Bus: MultirotorGuidanceControlBus
      link override EnvironmentSignalSpecification: OutDataTypeStr=Bus: MultirotorGuidanceEnvironmentBus
      link override State: BusOutputAsStruct=off
  TR_Pitch : Reshape  OutputDimensionality=Customize  OutputDimensions=[1 N_uav]
  TR_Roll : Reshape  OutputDimensionality=Customize  OutputDimensions=[1 N_uav]
  TR_Thrust : Reshape  OutputDimensionality=Customize  OutputDimensions=[1 N_uav]
  TR_YawRate : Reshape  OutputDimensionality=Customize  OutputDimensions=[1 N_uav]
  TransposeOri : Math  Operator=transpose
  TransposePos : Math  Operator=transpose
  TransposeVel : Math  Operator=transpose
  TruePos : Outport
  TrueVel : Outport  Port=2
  TrueOri : Outport  Port=3
  wires:
  CmdThrust/1 -> TR_Thrust/1
  CmdYawRate/1 -> TR_YawRate/1
  Gravity/1 -> EnvBus/1  "Gravity"
  CmdPitch/1 -> TR_Pitch/1
  CmdRoll/1 -> TR_Roll/1
  TR_Pitch/1 -> ControlBus/2  "Pitch"
  TR_Roll/1 -> ControlBus/1  "Roll"
  TR_Thrust/1 -> ControlBus/4  "Thrust"
  TR_YawRate/1 -> ControlBus/3  "YawRate"
  Bus Selector/1 -> TransposePos/1  "<WorldPosition>"
  ControlBus/1 -> GuidanceModel/1
  EnvBus/1 -> GuidanceModel/2
  Bus Selector/2 -> TransposeVel/1  "<WorldVelocity>"
  GuidanceModel/1 -> Bus Selector/1  "StateBus"
  Bus Selector/3 -> TransposeOri/1  "<EulerZYX>"
  TransposePos/1 -> TruePos/1
  TransposeVel/1 -> TrueVel/1
  TransposeOri/1 -> TrueOri/1

== system MultiUAV_DroneShow/DroneFleet/MissionStatus ==
  RxStatus : Inport
  AllComplete : MinMax
  ArrCount : UnitDelay  InitialCondition=uint32(0)  SampleTime=Ts_sim
  ArrGeTotal : RelationalOperator
  ArrSum : Sum  Inputs=|++  OutDataTypeStr=uint32  SaturateOnIntegerOverflow=on
  BoolToDbl : DataTypeConversion  OutDataTypeStr=double
  C_num_wp : Constant  Value=num_waypoints  OutDataTypeStr=double
  CmpComplete : RelationalOperator  Operator===
  DTC_ArrStatus : DataTypeConversion  OutDataTypeStr=uint32
  DTC_FlagsDbl : DataTypeConversion  OutDataTypeStr=double
  FlagsMat : Reshape  OutputDimensionality=Customize  OutputDimensions=[num_waypoints, N_uav]
  ReadFlags : DataStoreRead  DataStoreName=ReceivedFlags  IndexOptions=Index vector (dialog)  Indices=1  OutputSizes=1
  SumPerDrone : Sum  Inputs=1  CollapseMode=Specified dimension
  TotalItems : Constant  Value=uint32(N_uav*num_waypoints)  OutDataTypeStr=uint32
  UploadCount : Outport
  AllAccepted : Outport  Port=2
  MissionFlags : Outport  Port=3
  AckTrigger : Outport  Port=4
  wires:
  RxStatus/1 -> DTC_ArrStatus/1
  TotalItems/1 -> ArrGeTotal/2
  BoolToDbl/1 -> AckTrigger/1
  ReadFlags/1 -> FlagsMat/1
  FlagsMat/1 -> MissionFlags/1, DTC_FlagsDbl/1  "dbg_flags"
  DTC_ArrStatus/1 -> ArrSum/1
  ArrSum/1 -> ArrCount/1  "arr_count_next"
  DTC_FlagsDbl/1 -> SumPerDrone/1
  ArrCount/1 -> UploadCount/1, ArrGeTotal/1, ArrSum/2
  SumPerDrone/1 -> CmpComplete/1  "accepted_per_drone"
  C_num_wp/1 -> CmpComplete/2
  ArrGeTotal/1 -> BoolToDbl/1
  CmpComplete/1 -> AllComplete/1
  AllComplete/1 -> AllAccepted/1

== system MultiUAV_DroneShow/DroneFleet/Navigation ==
  TruePos : Inport
  TrueVel : Inport  Port=2
  TrueOri : Inport  Port=3
  PosSigma : Inport  Port=4
  AddGNSSErr : Sum  Inputs=|++
  BiasScale : Product
  FixAlwaysTrue : Constant  Value=true(N_uav,1)  OutDataTypeStr=boolean  SampleTime=Ts_sim
  GnssNoise : RandomNumber  Mean=zeros(N_uav,3)  Variance=ones(N_uav,3)  Seed=gnss_err_seed  SampleTime=Ts_sim
  INS : sensorinslib/INS  MountingLocation=[0 0 0]  RollAccuracy=0.003491  PitchAccuracy=0.003491  YawAccuracy=0.017453  PositionAccuracy=0.02  VelocityAccuracy=gps_vel_accuracy  UseAccelAndAngVel=off  AccelerationAccuracy=0  AngularVelocityAccuracy=0  TimeInput=on  PositionErrorFactor=[0.5 0.5 0.5]  SeedDouble=67  SimulateUsing=Code generation
      settings: LibrarySourceBlock=uavsimlib/INS
  LogINSPos : ToWorkspace  VariableName=insPositions  SaveFormat=Timeseries  SampleTime=-1
  NoiseDelay : UnitDelay  SampleTime=Ts_sim
  NoiseGainA : Gain  Gain=gnss_err_pole
  NoiseGainB : Gain  Gain=gnss_err_gain
  NoiseSum : Sum  Inputs=++|
  SigmaCat : Concatenate  NumInputs=3  Mode=Multidimensional array  ConcatenateDimension=2
  SigmaCol : Reshape  OutputDimensionality=Customize  OutputDimensions=[N_uav 1]
  EstVel : Outport
  EstOri : Outport  Port=2
  MeasPos : Outport  Port=3
  wires:
  TrueVel/1 -> INS/2
  TruePos/1 -> INS/1
  INS/3 -> EstOri/1
  SigmaCol/1 -> SigmaCat/2, SigmaCat/3, SigmaCat/1
  GnssNoise/1 -> NoiseGainB/1
  PosSigma/1 -> SigmaCol/1
  NoiseSum/1 -> NoiseDelay/1, BiasScale/1  "gnss_noise"
  SigmaCat/1 -> BiasScale/2
  TrueOri/1 -> INS/3
  FixAlwaysTrue/1 -> INS/4
  NoiseDelay/1 -> NoiseGainA/1
  INS/2 -> EstVel/1
  NoiseGainA/1 -> NoiseSum/1
  AddGNSSErr/1 -> MeasPos/1, LogINSPos/1  "meas_pos"
  NoiseGainB/1 -> NoiseSum/2
  BiasScale/1 -> AddGNSSErr/1
  INS/1 -> AddGNSSErr/2

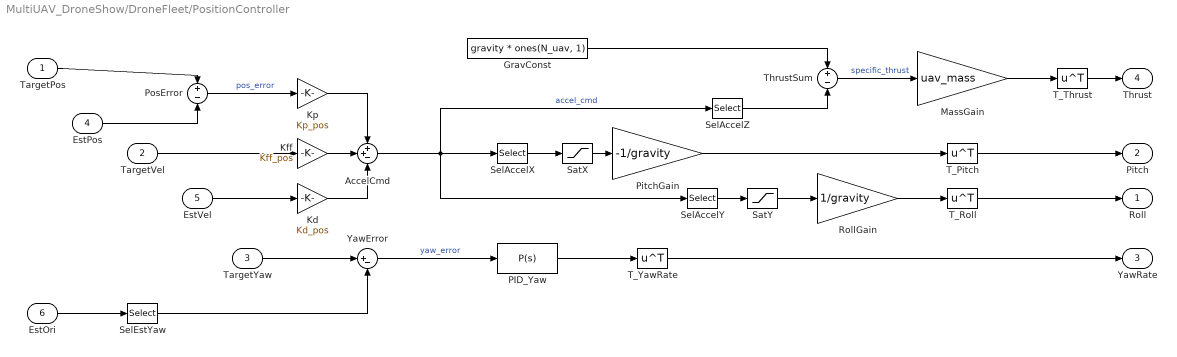
== system MultiUAV_DroneShow/DroneFleet/PositionController ==
  TargetPos : Inport
  TargetVel : Inport  Port=2
  TargetYaw : Inport  Port=3
  EstPos : Inport  Port=4
  EstVel : Inport  Port=5
  EstOri : Inport  Port=6
  AccelCmd : Sum  Inputs=++-
  GravConst : Constant  Value=gravity * ones(N_uav, 1)
  Kd : Gain  Gain=Kd_pos
  Kff : Gain  Gain=Kff_pos
  Kp : Gain  Gain=Kp_pos
  MassGain : Gain  Gain=uav_mass
  PID_Yaw : slpidlib/PID Controller  Controller=P  Form=Parallel  TimeDomain=Continuous-time  UseExternalTs=off  SampleTime=-1  IntegratorMethod=Forward Euler  FilterMethod=Forward Euler  ControllerParametersSource=internal  P=2.0  I=1  UseKiTs=off  D=0  UseExternalDerivativeSource=off  N=100  UseFilter=on  TunerSelectOption=Transfer Function Based (PID Tuner App)  InitialConditionSource=internal  InitialConditionForIntegrator=0  InitialConditionForFilter=0  DifferentiatorICPrevScaledInput=0  ExternalReset=none  TrackingMode=off  Kt=1  LimitOutput=on  SatLimitsSource=internal  UpperSaturationLimit=2.0  LowerSaturationLimit=-2.0  LinearizeAsGain=on  AntiWindupMode=none  Kb=1  LimitIntegrator=off  UpperIntegratorSaturationLimit=inf  LowerIntegratorSaturationLimit=-inf  POutMin=[]  POutMax=[]  IOutMin=[]  IOutMax=[]  DOutMin=[]  DOutMax=[]  NOutMin=[]  NOutMax=[]  SumOutMin=[]  SumOutMax=[]  SaturationOutMin=[]  SaturationOutMax=[]  PParamMin=[]  PParamMax=[]  IParamMin=[]  IParamMax=[]  DParamMin=[]  DParamMax=[]  NParamMin=[]  NParamMax=[]  KbParamMin=[]  KbParamMax=[]  KtParamMin=[]  KtParamMax=[]  KbOutMin=[]  KbOutMax=[]  KtOutMin=[]  KtOutMax=[]  IntegratorOutMin=[]  IntegratorOutMax=[]  FilterOutMin=[]  FilterOutMax=[]  SumI1OutMin=[]  SumI1OutMax=[]  SumI2OutMin=[]  SumI2OutMax=[]  SumI3OutMin=[]  SumI3OutMax=[]  SumI4OutMin=[]  SumI4OutMax=[]  SumDOutMin=[]  SumDOutMax=[]  DifferentiatorOutMin=[]  DifferentiatorOutMax=[]  FilterDiffOutCoefMin=[]  FilterDiffOutCoefMax=[]  ReciprocalOutMin=[]  ReciprocalOutMax=[]  SumDenOutMin=[]  SumDenOutMax=[]  SumNumOutMin=[]  SumNumOutMax=[]  DivideOutMin=[]  DivideOutMax=[]  UdiffTsProdOutMin=[]  UdiffTsProdOutMax=[]  NTsProdOutMin=[]  NTsProdOutMax=[]  UintegralTsProdOutMin=[]  UintegralTsProdOutMax=[]  UngainTsProdOutMin=[]  UngainTsProdOutMax=[]  ClampingZeroOutDataTypeStr=Inherit: Inherit via back propagation  ClampingZeroOutMin=[]  ClampingZeroOutMax=[]  FilterDenConstantOutDataTypeStr=Inherit: Inherit via back propagation  FilterDenConstantOutMin=[]  FilterDenConstantOutMax=[]  PCopyOutDataTypeStr=Inherit: Inherit via back propagation  PCopyOutMin=[]  PCopyOutMax=[]  NCopyOutDataTypeStr=Inherit: Inherit via back propagation  NCopyOutMin=[]  NCopyOutMax=[]  IntegratorContinuousStateAttributes=''  IntegratorStateMustResolveToSignalObject=off  IntegratorRTWStateStorageClass=Auto  FilterContinuousStateAttributes=''  FilterStateMustResolveToSignalObject=off  FilterRTWStateStorageClass=Auto  ParallelPVariant=InternalParameters  IdealPVariant=Disabled  IVariant=Disabled  DVariant=Disabled  IntegratorVariant=Disabled  SatVariant=Enabled  AWVariant=Disabled  PCopyVariant=Disabled  TRVariant=Disabled  FdbkBlocksVariant=Forward  IdealPFdbkVariant=Disabled  SatFdbkVariant=Disabled  DerivativeFilterVariant=Disabled  NVariant=Disabled  NCopyVariant=Disabled_SignalSpec  FilterICVariant=Disabled  IntegratorICVariant=Disabled  ExternalResetVariant=Disabled  TRSumVariant=Passthrough  SumFdbkVariant=Disabled  SumVariant=Passthrough_P  TsampFilterVariant=InternalTs  TsampNgainVariant=Passthrough  TsampIntegralVariant=Disabled_SignalSpec  ExternalSaturationOutDataTypeStr=Inherit: Same as second input  DerivativeSourceVariant=Disabled  PreIntVariant=InternalPreInt
  PitchGain : Gain  Gain=-1/gravity
  PosError : Sum  Inputs=+-
  RollGain : Gain  Gain=1/gravity
  SatX : Saturate  UpperLimit=3.0  LowerLimit=-3.0
  SatY : Saturate  UpperLimit=3.0  LowerLimit=-3.0
  SelAccelX : Selector  NumberOfDimensions=2  InputPortWidth=3  IndexOptions=Select all,Index vector (dialog)  Indices=1,1  OutputSizes=1,1
  SelAccelY : Selector  NumberOfDimensions=2  InputPortWidth=3  IndexOptions=Select all,Index vector (dialog)  Indices=1,2  OutputSizes=1,1
  SelAccelZ : Selector  NumberOfDimensions=2  InputPortWidth=3  IndexOptions=Select all,Index vector (dialog)  Indices=1,3  OutputSizes=1,1
  SelEstYaw : Selector  NumberOfDimensions=2  InputPortWidth=3  IndexOptions=Select all,Index vector (dialog)  Indices=1,3  OutputSizes=1,1
  T_Pitch : Math  Operator=transpose
  T_Roll : Math  Operator=transpose
  T_Thrust : Math  Operator=transpose
  T_YawRate : Math  Operator=transpose
  ThrustSum : Sum  Inputs=+-
  YawError : Sum  Inputs=|+-
  Roll : Outport
  Pitch : Outport  Port=2
  YawRate : Outport  Port=3
  Thrust : Outport  Port=4
  wires:
  T_Thrust/1 -> Thrust/1
  T_Roll/1 -> Roll/1
  T_Pitch/1 -> Pitch/1
  T_YawRate/1 -> YawRate/1
  ThrustSum/1 -> MassGain/1  "specific_thrust"
  PID_Yaw/1 -> T_YawRate/1
  SelAccelZ/1 -> ThrustSum/2
  GravConst/1 -> ThrustSum/1
  RollGain/1 -> T_Roll/1
  YawError/1 -> PID_Yaw/1  "yaw_error"
  SelEstYaw/1 -> YawError/2
  TargetYaw/1 -> YawError/1
  EstOri/1 -> SelEstYaw/1
  PosError/1 -> Kp/1  "pos_error"
  PitchGain/1 -> T_Pitch/1
  TargetPos/1 -> PosError/1
  EstPos/1 -> PosError/2
  MassGain/1 -> T_Thrust/1
  AccelCmd/1 -> SelAccelZ/1, SelAccelX/1, SelAccelY/1  "accel_cmd"
  SelAccelX/1 -> SatX/1
  SatX/1 -> PitchGain/1
  SelAccelY/1 -> SatY/1
  SatY/1 -> RollGain/1
  Kp/1 -> AccelCmd/1
  TargetVel/1 -> Kff/1
  Kff/1 -> AccelCmd/2
  EstVel/1 -> Kd/1
  Kd/1 -> AccelCmd/3

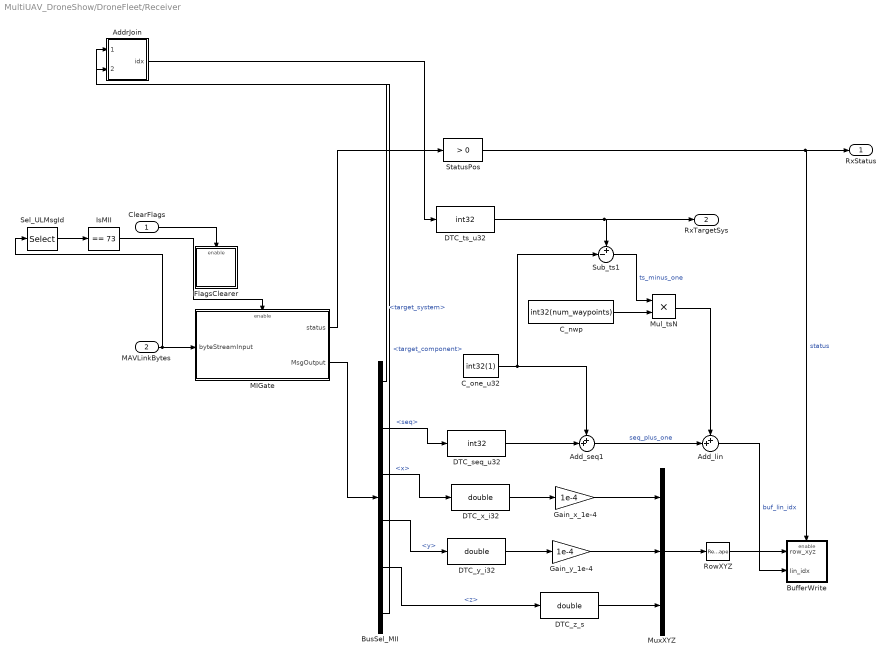
== system MultiUAV_DroneShow/DroneFleet/Receiver ==
  ClearFlags : Inport
  MAVLinkBytes : Inport  Port=2
  Add_lin : Sum  Inputs=++|  OutDataTypeStr=int32
  Add_seq1 : Sum  Inputs=++|  OutDataTypeStr=int32
  AddrJoin : Subsystem
  BufferWrite : Subsystem
  BusSel_MII : BusSelector  OutputSignals=Payload.target_system,Payload.seq,Payload.x,Payload.y,Payload.z,Payload.target_component
  C_nwp : Constant  Value=int32(num_waypoints)  OutDataTypeStr=int32
  C_one_u32 : Constant  Value=int32(1)  OutDataTypeStr=int32
  DTC_seq_u32 : DataTypeConversion  OutDataTypeStr=int32
  DTC_ts_u32 : DataTypeConversion  OutDataTypeStr=int32
  DTC_x_i32 : DataTypeConversion  OutDataTypeStr=double
  DTC_y_i32 : DataTypeConversion  OutDataTypeStr=double
  DTC_z_s : DataTypeConversion  OutDataTypeStr=double
  FlagsClearer : Subsystem  TreatAsAtomicUnit=on
  Gain_x_1e-4 : Gain  Gain=1e-4
  Gain_y_1e-4 : Gain  Gain=1e-4
  IsMII : simulink/Logic and Bit Operations/Compare To Constant  relop===  const=73  OutDataTypeStr=boolean
  MIGate : Subsystem
  Mul_tsN : Product  OutDataTypeStr=int32
  MuxXYZ : Mux  Inputs=3
  RowXYZ : Reshape  OutputDimensionality=Customize  OutputDimensions=[1 3]
  Sel_ULMsgId : Selector  NumberOfDimensions=2  InputPortWidth=3  IndexOptions=Index vector (dialog),Index vector (dialog)  Indices=1,8  OutputSizes=1,1
  StatusPos : hdlsllib/Logic and Bit Operations/Compare To Constant  relop=>  const=0  OutDataTypeStr=boolean
  Sub_ts1 : Sum  Inputs=+-|  OutDataTypeStr=int32
  RxStatus : Outport
  RxTargetSys : Outport  Port=2
  wires:
  ClearFlags/1 -> FlagsClearer/Enable
  StatusPos/1 -> RxStatus/1, BufferWrite/Enable  "status"
  BusSel_MII/2 -> DTC_seq_u32/1  "<seq>"
  DTC_z_s/1 -> MuxXYZ/3
  Sub_ts1/1 -> Mul_tsN/1  "ts_minus_one"
  BusSel_MII/3 -> DTC_x_i32/1  "<x>"
  BusSel_MII/4 -> DTC_y_i32/1  "<y>"
  BusSel_MII/5 -> DTC_z_s/1  "<z>"
  DTC_ts_u32/1 -> RxTargetSys/1, Sub_ts1/1
  DTC_seq_u32/1 -> Add_seq1/2
  C_one_u32/1 -> Sub_ts1/2, Add_seq1/1
  DTC_x_i32/1 -> Gain_x_1e-4/1
  DTC_y_i32/1 -> Gain_y_1e-4/1
  C_nwp/1 -> Mul_tsN/2
  Mul_tsN/1 -> Add_lin/1
  Add_seq1/1 -> Add_lin/2  "seq_plus_one"
  Gain_x_1e-4/1 -> MuxXYZ/1
  Gain_y_1e-4/1 -> MuxXYZ/2
  MuxXYZ/1 -> RowXYZ/1
  Add_lin/1 -> BufferWrite/2(lin_idx)  "buf_lin_idx"
  RowXYZ/1 -> BufferWrite/1(row_xyz)
  MAVLinkBytes/1 -> MIGate/1(byteStreamInput), Sel_ULMsgId/1
  MIGate/1(status) -> StatusPos/1
  MIGate/2(MsgOutput) -> BusSel_MII/1
  Sel_ULMsgId/1 -> IsMII/1
  IsMII/1 -> MIGate/Enable
  BusSel_MII/1 -> AddrJoin/1(target_system)  "<target_system>"
  BusSel_MII/6 -> AddrJoin/2(target_component)  "<target_component>"
  AddrJoin/1(idx) -> DTC_ts_u32/1

== system MultiUAV_DroneShow/DroneFleet/SetpointGenerator ==
  LandNow : Inport
  ShowTime : Inport  Port=2
  LandingOverride : Subsystem
  PlannedTrajectory : Subsystem
  CmdPos : Outport
  CmdVel : Outport  Port=2
  CmdYaw : Outport  Port=3
  wires:
  ShowTime/1 -> PlannedTrajectory/1(ShowTime)  "show_time"
  LandingOverride/2(CmdVel) -> CmdVel/1
  PlannedTrajectory/2(PlanVel) -> LandingOverride/3(PlanVel)
  PlannedTrajectory/1(PlanPos) -> LandingOverride/2(PlanPos)
  PlannedTrajectory/3(PlanYaw) -> CmdYaw/1
  LandNow/1 -> LandingOverride/1(LandNow)
  LandingOverride/1(CmdPos) -> CmdPos/1

== system MultiUAV_DroneShow/DroneFleet/Transmitter ==
  MissionFlags : Inport
  AckTrigger : Inport  Port=2
  RxStatus : Inport  Port=3
  RxTargetSys : Inport  Port=4
  EstVel : Inport  Port=5
  MeasPos : Inport  Port=6
  DownlinkMux : Subsystem
  MissionAckEncoder : Subsystem
  MissionRequestEncoder : Subsystem
  TelemetryCat : Concatenate  Mode=Multidimensional array  ConcatenateDimension=2
  TelemetryEncoder : Subsystem
  TelemetryTxEnable : Constant  Value=telemetry_tx_enable  SampleTime=Ts_sim
  TelemetryBus : Outport
  MAVLinkBytes : Outport  Port=2
  wires:
  EstVel/1 -> TelemetryEncoder/1(EstVel), TelemetryCat/2
  RxTargetSys/1 -> MissionRequestEncoder/1(RxTargetSys)
  MissionFlags/1 -> MissionRequestEncoder/2(MissionFlags)
  RxStatus/1 -> MissionRequestEncoder/3(RxStatus)
  AckTrigger/1 -> MissionAckEncoder/1(AckTrigger)
  MeasPos/1 -> TelemetryEncoder/2(MeasPos), TelemetryCat/1
  MissionRequestEncoder/1(ReqBytes) -> DownlinkMux/1(ReqBytes)
  DownlinkMux/1(MAVLinkBytes) -> MAVLinkBytes/1
  MissionRequestEncoder/2(ReqPending) -> DownlinkMux/2(ReqPending)
  MissionAckEncoder/1(AckBytes) -> DownlinkMux/3(AckBytes)
  MissionAckEncoder/2(AckActive) -> DownlinkMux/4(AckActive)
  TelemetryEncoder/1(TelemetryBytes) -> DownlinkMux/5(TelemetryBytes)
  TelemetryCat/1 -> TelemetryBus/1
  TelemetryTxEnable/1 -> TelemetryEncoder/Enable
